simulink model "rotation_block"  (R2017b)
settings: Solver=VariableStepAuto  StartTime=0.0  StopTime=10.0  RelTol=1e-3

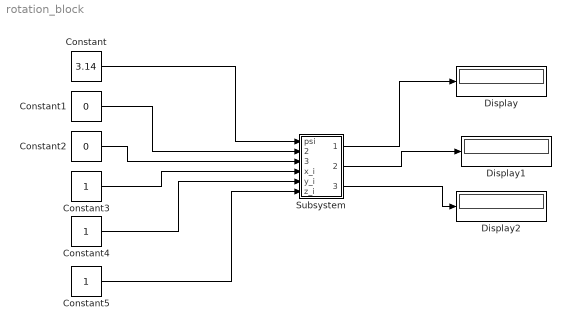
== system rotation_block ==
  Constant : Constant  Value=3.14
  Constant1 : Constant  Value=0
  Constant2 : Constant  Value=0
  Constant3 : Constant
  Constant4 : Constant
  Constant5 : Constant
  Display : Display
  Display1 : Display
  Display2 : Display
  Subsystem : Subsystem
  wires:
  Constant/1 -> Subsystem/1(psi)
  Constant1/1 -> Subsystem/2(theta)
  Constant2/1 -> Subsystem/3(phi)
  Constant3/1 -> Subsystem/4("x_i ")
  Constant4/1 -> Subsystem/5(y_i)
  Constant5/1 -> Subsystem/6(z_i)
  Subsystem/1(x_b) -> Display/1
  Subsystem/2(y_b) -> Display1/1
  Subsystem/3(z_b) -> Display2/1

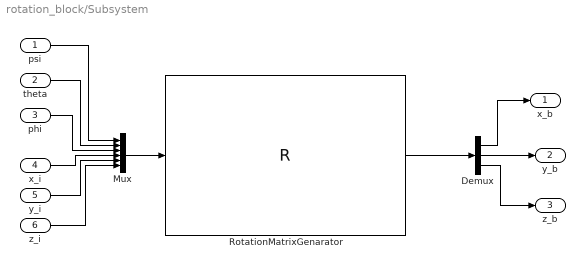
== system rotation_block/Subsystem ==
  psi : Inport  OutMin=-pi  OutMax=pi
  theta : Inport  Port=2  OutMin=0  OutMax=0
  phi : Inport  Port=3  OutMin=0  OutMax=0
  "x_i " : Inport  Port=4  OutMin=0  OutMax=0
  y_i : Inport  Port=5  OutMin=1  OutMax=1
  z_i : Inport  Port=6  OutMin=1  OutMax=1
  Demux : Demux  Outputs=3
  Mux : Mux  Inputs=6
  RotationMatrixGenarator : MATLABFcn  MATLABFcn=R
  x_b : Outport
  y_b : Outport  Port=2
  z_b : Outport  Port=3
  wires:
  phi/1 -> Mux/3
  psi/1 -> Mux/1
  Mux/1 -> RotationMatrixGenarator/1
  theta/1 -> Mux/2
  y_i/1 -> Mux/5
  z_i/1 -> Mux/6
  "x_i "/1 -> Mux/4
  Demux/2 -> y_b/1
  RotationMatrixGenarator/1 -> Demux/1
  Demux/3 -> z_b/1
  Demux/1 -> x_b/1
